simulink model "makeFigs"  (R2019a)
settings: Solver=VariableStepAuto  StartTime=0.0  StopTime=70  RelTol=1e-2
values from neighbouring files (symbols this model uses):
  A = 1/JT *[zeros(2,2),JT*eye(2,2);     0 ,1/4 * mp^2 *Lp^2*Lr*g, -(Jp + 1/4 *mp*Lp^2)*Dr, -1/2*mp*Lr*Lp*Dp;     0,1/2 *mp*Lp*g*(Jr + mp*Lr^2),-1/2*mp*Lp*Lr*Dr, -(Jr +mp*Lr^2)*Dp]    [dp2script.m]    (also in jacobA.m = [0,0,1,0;0,0,0,1;0,Lp.*mp.*Rm.^(-1).*((-4).*Lp.^2.*Lr.^2.*mp)
  B = ng*nm*Kg*Kt /Rm *B    [dp2script.m]    (also in jacobA.m = [0;0;4.*Kg.*Kt.*(4.*Jp+Lp.^2.*mp).*n.*Rm.^(-1).*((-4).*Lp.^2; nonLinear.m = [(tau-Dr*dtheta); -Dp*dalpha])
  C = eye(2,4)    [dp2script.m]    (also in nonLinear.m = [A3, A4;B3,0])
  g = 9.81    [dp2script.m]    (also in jacobA.m; nonLinear.m)
  Jp = 0.0012    [dp2script.m]    (also in jacobA.m; nonLinear.m)
  Jr = 0.0020    (= 0.002)    [dp2script.m]    (also in jacobA.m; nonLinear.m)
  K = place(A,B,p)    [dp2script.m]    (also in placeA.m = Bv(:,1:m) * K)
  Kg = 70    [dp2script.m]    (also in jacobA.m; nonLinear.m)
  km = 7.68e-3    (= 0.00768)    [dp2script.m]    (also in jacobA.m; nonLinear.m)
  Kt = 7.68e-3    (= 0.00768)    [dp2script.m]    (also in jacobA.m; nonLinear.m)
  L = place(A',C',[-4,-4.5,-5,-5.5])'    [dp2script.m]    (also in placeA.m = L.')
  Lp = 0.129    [dp2script.m]    (also in jacobA.m; nonLinear.m)
  Lr = 0.085    [dp2script.m]    (also in jacobA.m; nonLinear.m)
  mp = 0.127    [dp2script.m]    (also in jacobA.m; nonLinear.m)
  n = ng*nm    (= 0.621)    [dp2script.m]    (also in jacobA.m; nonLinear.m)
  Rm = 8.40    (= 8.4)    [dp2script.m]    (also in jacobA.m; nonLinear.m)
libraries: simulink x2
settings Model: Creator=Ankith A Das  LastModifiedBy=Ankith A Das

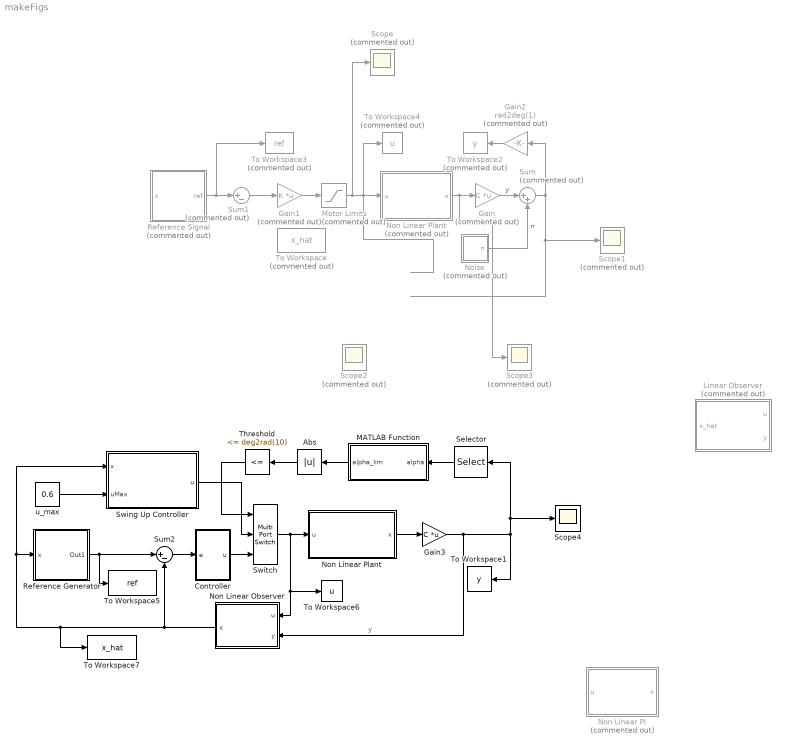
== system makeFigs ==
  Abs : Abs
  Controller : Subsystem
  Gain : Gain  Commented=on  Gain=C  Multiplication=Matrix(K*u)
  Gain1 : Gain  Commented=on  Gain=K  Multiplication=Matrix(K*u)
  Gain2 : Gain  Commented=on  Gain=rad2deg(1)
  Gain3 : Gain  Gain=C  Multiplication=Matrix(K*u)
  Linear Observer : Subsystem  Commented=on
  MATLAB Function : MATLAB Function  TreatAsAtomicUnit=on
  Motor Limits : Saturate  Commented=on  UpperLimit=6  LowerLimit=-6
  Noise : Subsystem  Commented=on
  Non Linear Observer : Subsystem
  "Non Linear Pl " : Subsystem  Commented=on
  Non Linear Plant : Subsystem  Commented=on
  "Non Linear Plant " : Subsystem
  Reference Generator : Subsystem
  Reference Signal : Subsystem  Commented=on
  Scope{,1..3} (4 alike) : Scope  Commented=on
  Scope4 : Scope
  Selector : Selector  InputPortWidth=2  IndexOptions=Index vector (dialog)  Indices=[2]  OutputSizes=1
  Sum : Sum  Commented=on  Inputs=|++
  Sum1 : Sum  Commented=on  Inputs=|+-
  Sum2 : Sum  Inputs=|+-
  Swing Up Controller : Subsystem
  Switch : MultiPortSwitch  DataPortOrder=Zero-based contiguous  Inputs=2  zeroidx=on
  Threshold : simulink/Logic and Bit Operations/Compare To Constant  relop=<=  const=deg2rad(10)  OutDataTypeStr=uint8
  To Workspace : ToWorkspace  Commented=on  VariableName=x_hat  SaveFormat=Structure With Time  SampleTime=-1
  To Workspace1 : ToWorkspace  VariableName=y  SaveFormat=Structure With Time  SampleTime=-1
  To Workspace2 : ToWorkspace  Commented=on  VariableName=y  SaveFormat=Structure With Time  SampleTime=-1
  To Workspace3 : ToWorkspace  Commented=on  VariableName=ref  SaveFormat=Structure  SampleTime=-1
  To Workspace4 : ToWorkspace  Commented=on  VariableName=u  SaveFormat=Structure  SampleTime=-1
  To Workspace5 : ToWorkspace  VariableName=ref  SaveFormat=Structure  SampleTime=-1
  To Workspace6 : ToWorkspace  VariableName=u  SaveFormat=Structure  SampleTime=-1
  To Workspace7 : ToWorkspace  VariableName=x_hat  SaveFormat=Timeseries  SampleTime=-1
  u_max : Constant  Value=0.6
  wires:
  Reference Signal/1(ref) -> To Workspace3/1, Sum1/1
  Gain2/1 -> To Workspace2/1
  Non Linear Plant/1(x) -> Scope3/1, Gain/1
  Gain1/1 -> Motor Limits/1
  Sum1/1 -> Gain1/1
  Motor Limits/1 -> Scope/1, To Workspace4/1, Non Linear Plant/1(u)
  Sum/1 -> Scope1/1, Gain2/1
  Gain/1 -> Sum/1  "y"
  Noise/1("n ") -> Sum/2  "n"
  ? -> Scope2/1, To Workspace/1, Reference Signal/1(x), Sum1/2
  Controller/1(u) -> Switch/3
  Abs/1 -> Threshold/1
  Reference Generator/1(Out1) -> To Workspace5/1, Sum2/1
  Threshold/1 -> Switch/1
  Swing Up Controller/1(u) -> Switch/2
  u_max/1 -> Swing Up Controller/2(uMax)
  Switch/1 -> Non Linear Observer/1(u), To Workspace6/1, "Non Linear Plant "/1(u)
  MATLAB Function/1(alpha_lim) -> Abs/1
  "Non Linear Plant "/1(x) -> Gain3/1
  Gain3/1 -> Non Linear Observer/2(y), To Workspace1/1, Scope4/1, Selector/1  "y"
  Sum2/1 -> Controller/1(e)
  Selector/1 -> MATLAB Function/1(alpha)
  Non Linear Observer/1(x) -> Sum2/2, To Workspace7/1, Swing Up Controller/1(x), Reference Generator/1(x)

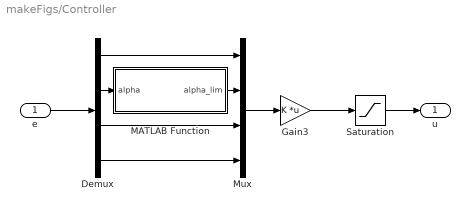
== system makeFigs/Controller ==
  e : Inport
  Demux : Demux
  Gain3 : Gain  Gain=K  Multiplication=Matrix(K*u)
  MATLAB Function : MATLAB Function  TreatAsAtomicUnit=on
  Mux : Mux
  Saturation : Saturate  UpperLimit=6  LowerLimit=-6
  u : Outport
  wires:
  e/1 -> Demux/1
  Demux/1 -> Mux/1
  Demux/4 -> Mux/4
  Demux/2 -> MATLAB Function/1(alpha)
  Demux/3 -> Mux/3
  MATLAB Function/1(alpha_lim) -> Mux/2
  Mux/1 -> Gain3/1
  Gain3/1 -> Saturation/1
  Saturation/1 -> u/1

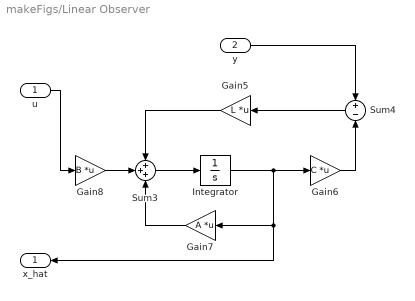
== system makeFigs/Linear Observer ==
  u : Inport
  y : Inport  Port=2
  Gain5 : Gain  Gain=L  Multiplication=Matrix(K*u)
  Gain6 : Gain  Gain=C  Multiplication=Matrix(K*u)
  Gain7 : Gain  Gain=A  Multiplication=Matrix(K*u)
  Gain8 : Gain  Gain=B  Multiplication=Matrix(K*u)
  Integrator : Integrator  InitialCondition=[0,0,0,0]'
  Sum3 : Sum  Inputs=+++
  Sum4 : Sum  Inputs=+|-
  x_hat : Outport
  wires:
  Gain6/1 -> Sum4/2
  Integrator/1 -> x_hat/1, Gain7/1, Gain6/1
  Gain5/1 -> Sum3/1
  Gain7/1 -> Sum3/3
  Sum3/1 -> Integrator/1
  y/1 -> Sum4/1
  Gain8/1 -> Sum3/2
  Sum4/1 -> Gain5/1
  u/1 -> Gain8/1

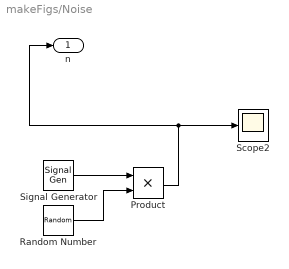
== system makeFigs/Noise ==
  Product : Product
  Random Number : RandomNumber  SampleTime=0.1
  Scope2 : Scope
  Signal Generator : SignalGenerator  Amplitude=0.015  Frequency=2900  Units=rad/sec
  "n " : Outport
  wires:
  Signal Generator/1 -> Product/1
  Product/1 -> "n "/1, Scope2/1
  Random Number/1 -> Product/2

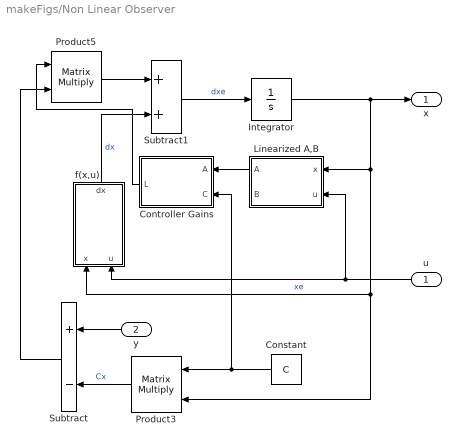
== system makeFigs/Non Linear Observer ==
  u : Inport
  y : Inport  Port=2
  Constant : Constant  Value=C
  Controller Gains : MATLAB Function  TreatAsAtomicUnit=on
  Integrator : Integrator  InitialCondition=[0.5,0.5,0,0]'
  Linearized A,B : MATLAB Function  TreatAsAtomicUnit=on
  Product3 : Product  SCDEnableBlockLinearizationSpecification=on  Multiplication=Matrix(*)
  Product5 : Product  SCDEnableBlockLinearizationSpecification=on  Multiplication=Matrix(*)
  Subtract : Sum  Inputs=+-
  Subtract1 : Sum
  f(x,u) : MATLAB Function  TreatAsAtomicUnit=on
  x : Outport
  wires:
  Subtract1/1 -> Integrator/1  "dxe"
  y/1 -> Subtract/1
  Controller Gains/1(L) -> Product5/1
  Subtract/1 -> Product5/2
  Product5/1 -> Subtract1/1
  Constant/1 -> Product3/1, Controller Gains/2(C)
  Product3/1 -> Subtract/2  "Cx"
  Integrator/1 -> x/1, Product3/2, f(x,u)/1(x), Linearized A,B/1(x)  "xe"
  u/1 -> f(x,u)/2(u), Linearized A,B/2(u)
  Linearized A,B/1(A) -> Controller Gains/1(A)
  f(x,u)/1(dx) -> Subtract1/2  "dx"

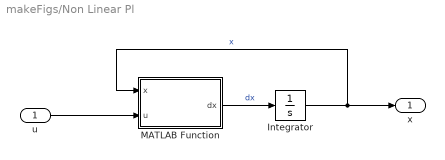
== system makeFigs/Non Linear Pl  ==
  u : Inport
  Integrator : Integrator  InitialCondition=[0,0,0,0]'
  MATLAB Function : MATLAB Function  TreatAsAtomicUnit=on
  x : Outport
  wires:
  Integrator/1 -> x/1, MATLAB Function/1(x)  "x"
  u/1 -> MATLAB Function/2(u)
  MATLAB Function/1(dx) -> Integrator/1  "dx"

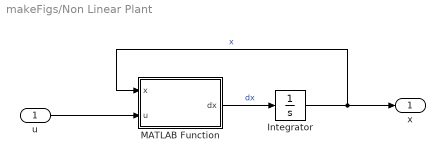
== system makeFigs/Non Linear Plant ==
  u : Inport
  Integrator : Integrator  InitialCondition=[0,0,0,0]'
  MATLAB Function : MATLAB Function  TreatAsAtomicUnit=on
  x : Outport
  wires:
  Integrator/1 -> x/1, MATLAB Function/1(x)  "x"
  u/1 -> MATLAB Function/2(u)
  MATLAB Function/1(dx) -> Integrator/1  "dx"

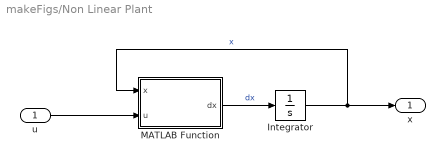
== system makeFigs/Non Linear Plant  ==
  u : Inport
  Integrator : Integrator  InitialCondition=[0,pi+0.5,0,0]'
  MATLAB Function : MATLAB Function  TreatAsAtomicUnit=on
  x : Outport
  wires:
  Integrator/1 -> x/1, MATLAB Function/1(x)  "x"
  u/1 -> MATLAB Function/2(u)
  MATLAB Function/1(dx) -> Integrator/1  "dx"

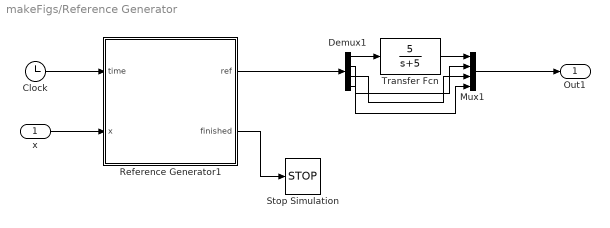
== system makeFigs/Reference Generator ==
  x : Inport
  Clock : Clock
  Demux1 : Demux
  Mux1 : Mux
  Reference Generator1 : MATLAB Function  TreatAsAtomicUnit=on  SystemSampleTime=0.002
  Stop Simulation : Stop
  Transfer Fcn : TransferFcn  Numerator=[5]  Denominator=[1 5]
  Out1 : Outport
  wires:
  Demux1/1 -> Transfer Fcn/1
  Mux1/1 -> Out1/1
  Demux1/4 -> Mux1/4
  Demux1/3 -> Mux1/3
  Demux1/2 -> Mux1/2
  x/1 -> Reference Generator1/2(x)
  Reference Generator1/1(ref) -> Demux1/1
  Reference Generator1/2(finished) -> Stop Simulation/1
  Transfer Fcn/1 -> Mux1/1
  Clock/1 -> Reference Generator1/1(time)

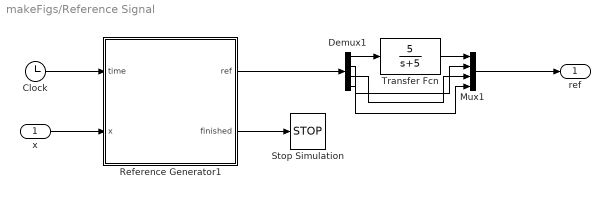
== system makeFigs/Reference Signal ==
  x : Inport
  Clock : Clock
  Demux1 : Demux
  Mux1 : Mux
  Reference Generator1 : MATLAB Function  TreatAsAtomicUnit=on  SystemSampleTime=0.002
  Stop Simulation : Stop
  Transfer Fcn : TransferFcn  Numerator=[5]  Denominator=[1 5]
  ref : Outport
  wires:
  Demux1/1 -> Transfer Fcn/1
  Mux1/1 -> ref/1
  Demux1/4 -> Mux1/4
  Demux1/3 -> Mux1/3
  Demux1/2 -> Mux1/2
  x/1 -> Reference Generator1/2(x)
  Reference Generator1/1(ref) -> Demux1/1
  Reference Generator1/2(finished) -> Stop Simulation/1
  Transfer Fcn/1 -> Mux1/1
  Clock/1 -> Reference Generator1/1(time)

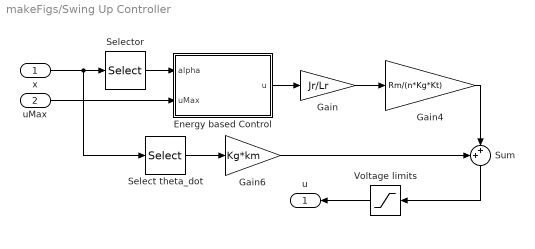
== system makeFigs/Swing Up Controller ==
  x : Inport
  uMax : Inport  Port=2
  Energy based Control : Subsystem
  Gain : Gain  Gain=Jr/Lr
  Gain4 : Gain  Gain=Rm/(n*Kg*Kt)
  Gain6 : Gain  Gain=Kg*km
  Select theta_dot : Selector  InputPortWidth=4  IndexOptions=Index vector (dialog)  Indices=[3]  OutputSizes=1
  Selector : Selector  InputPortWidth=4  IndexOptions=Index vector (dialog)  Indices=[2 4]  OutputSizes=1
  Sum : Sum  Inputs=++|
  Voltage limits : Saturate  UpperLimit=3  LowerLimit=-3
  u : Outport
  wires:
  Gain6/1 -> Sum/1
  Energy based Control/1(u) -> Gain/1
  Selector/1 -> Energy based Control/1(alpha)
  x/1 -> Select theta_dot/1, Selector/1
  Gain/1 -> Gain4/1
  Gain4/1 -> Sum/2
  uMax/1 -> Energy based Control/2("uMax ")
  Select theta_dot/1 -> Gain6/1
  Sum/1 -> Voltage limits/1
  Voltage limits/1 -> u/1

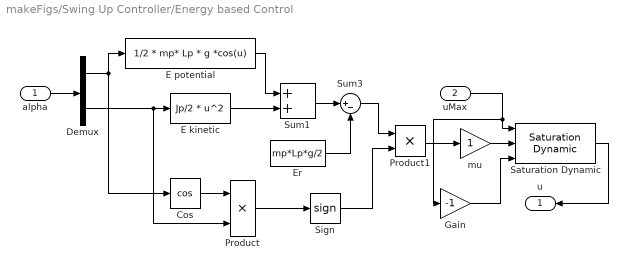
== system makeFigs/Swing Up Controller/Energy based Control ==
  alpha : Inport
  "uMax " : Inport  Port=2
  Cos : Trigonometry  Operator=cos
  Demux : Demux  Outputs=2
  E kinetic : Fcn  Expr=Jp/2 * u^2
  E potential : Fcn  Expr=1/2 * mp* Lp * g *cos(u)
  Er : Constant  Value=mp*Lp*g/2
  Gain : Gain  Gain=-1
  Product : Product
  Product1 : Product
  Saturation Dynamic : simulink/Discontinuities/Saturation Dynamic  OutMin=[]  OutMax=[]  OutDataTypeStr=Inherit: Same as second input  OutDataType=fixdt(1, 16)  OutScaling=2^-10  DoSatur=off
  Sign : Signum  ZeroCross=off
  Sum1 : Sum
  Sum3 : Sum  Inputs=|+-
  mu : Gain
  u : Outport
  wires:
  Sum1/1 -> Sum3/1
  Cos/1 -> Product/1
  Product/1 -> Sign/1
  Er/1 -> Sum3/2
  Product1/1 -> mu/1
  "uMax "/1 -> Saturation Dynamic/1, Gain/1
  Gain/1 -> Saturation Dynamic/3
  alpha/1 -> Demux/1
  mu/1 -> Saturation Dynamic/2
  Saturation Dynamic/1 -> u/1
  Sum3/1 -> Product1/1
  Sign/1 -> Product1/2
  Demux/2 -> E kinetic/1, Product/2
  E kinetic/1 -> Sum1/2
  E potential/1 -> Sum1/1
  Demux/1 -> Cos/1, E potential/1

== matlab function makeFigs/Non Linear Plant /MATLAB Function ==
  data: x input; u input; dx output
function dx = fullSystem(x,u)
    dx = nonLinear(x,u);
end

== matlab function makeFigs/Reference Generator/Reference Generator1 ==
  data: time input; x input size=4; ref output; finished output
function [ref, finished] = REFGEN(time, x)


persistent n 

persistent goodSteps 
persistent done
persistent recTime

if(isempty(n))
    n = 1; % start at first waypoint
    done = false;
end
if(isempty(goodSteps))
    goodSteps = 1;
end
if(isempty(recTime))
    recTime = -1; % start at first waypoint
end
    ref = zeros(4,1);
    x(2) = mod(x(2) + pi,2*pi)-pi;
    % Local variables
    waypoints = [30; -60; 45; -30]*pi/180; % reference waypoints
    posTolArm = 1*pi/180; % [rad] position tolerance
    posTolPend = posTolArm;
    velTolArm = 0.1; % [rad/s] velocity tolerance
    velTolPend = 0.1; % [rad/s] basically KF tolerance.

    if (abs(waypoints(n)-x(1)) <= posTolArm) && (abs(x(2)) <= posTolPend) && (abs(x(3)) <= velTolArm) && (abs(x(4)) <= velTolPend) % q1 and q2 stationary
        goodSteps = goodSteps + 1; % increment count if everything satisifed this timestep
        if recTime == -1
            recTime = time;
        end
    else
        goodSteps = 1; % reset if tolerances breached
        recTime = -1;
    end

    rst = false;
    %% detect successful completion of waypoint
    holdTime = 3;
    if time - recTime >= holdTime && recTime ~= -1
        rst = true;
        n = n + 1;
        if n > length(waypoints)
            done = true;
        end
        recTime = -1;
    end
%% Output reference
if(~done)
    ref(1) = waypoints(n);
    finished = done;
else
    ref(1) = waypoints(end);
    finished = done;
end

== matlab function makeFigs/Controller/MATLAB Function ==
  data: alpha input; alpha_lim output
function alpha_lim = fcn(alpha)
    alpha_lim = mod(alpha + pi,2*pi)-pi;
end

== matlab function makeFigs/MATLAB Function ==
  data: alpha input; alpha_lim output
function alpha_lim = fcn(alpha)
    alpha_lim = mod(alpha + pi,2*pi)-pi;
end

== matlab function makeFigs/Reference Signal/Reference Generator1 ==
  data: time input; x input size=4; ref output; finished output
function [ref, finished] = REFGEN(time, x)


persistent n 

persistent goodSteps 
persistent done
persistent recTime

if(isempty(n))
    n = 1; % start at first waypoint
    done = false;
end
if(isempty(goodSteps))
    goodSteps = 1;
end
if(isempty(recTime))
    recTime = -1; % start at first waypoint
end
    ref = zeros(4,1);
    x(2) = mod(x(2) + pi,2*pi)-pi;
    % Local variables
    waypoints = [30; -60; 45; -30]*pi/180; % reference waypoints
    posTolArm = 3*pi/180; % [rad] position tolerance
    posTolPend = posTolArm;
    velTolArm = 0.1; % [rad/s] velocity tolerance
    velTolPend = 0.1; % [rad/s] basically KF tolerance.

    if (abs(waypoints(n)-x(1)) <= posTolArm) && (abs(x(2)) <= posTolPend) && (abs(x(3)) <= velTolArm) && (abs(x(4)) <= velTolPend) % q1 and q2 stationary
        goodSteps = goodSteps + 1; % increment count if everything satisifed this timestep
        if recTime == -1
            recTime = time;
        end
    else
        goodSteps = 1; % reset if tolerances breached
        recTime = -1;
    end

    rst = false;
    %% detect successful completion of waypoint
    holdTime = 3;
    if time - recTime >= holdTime && recTime ~= -1
        rst = true;
        n = n + 1;
        if n > length(waypoints)
            done = true;
        end
        recTime = -1;
    end
%% Output reference
if(~done)
    ref(1) = waypoints(n);
    finished = done;
else
    ref(1) = waypoints(end);
    finished = done;
end

== matlab function makeFigs/Non Linear Observer/Linearized A,B ==
  data: x input; u input; A output; B output
function [A,B] = fcn(x,u)
    [A,B] = jacobA(x,u);
    
    %A = zeros(4,4);
    %B = zeros(4,1);
end

== matlab function makeFigs/Non Linear Plant/MATLAB Function ==
  data: x input; u input; dx output
function dx = fullSystem(x,u)
    dx = nonLinear(x,u);
end

== matlab function makeFigs/Non Linear Observer/Controller Gains ==
  data: A input; L output; C input
function L = fcn(A,C)
   L = placeA(A',C',[-4,-4.5,-5,-5.5]).';
end

== matlab function makeFigs/Non Linear Observer/f(x,u) ==
  data: x input; u input; dx output
function dx = fullSystem(x,u)
    dx = nonLinear(x,u);
end

== matlab function makeFigs/Non Linear Pl /MATLAB Function ==
  data: x input; u input; dx output
function dx = fullSystem(x,u)
    dx = nonLinear(x,u);
end
